simulink library "truetime"  (R2012a)
settings: Solver=ode45  SolverMode=SingleTasking  StartTime=0.0  StopTime=10.0  RelTol=1e-3
undefined symbols (not defined in the file or in its folder): sfunchk
settings Model: ExtModeAutoUpdateStatusClock=off  Creator=dan  LastModifiedBy=AC

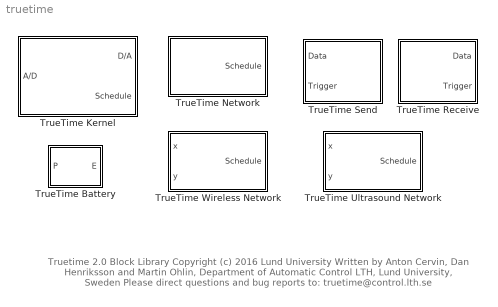
== system truetime ==
  note: Truetime 2.0  Block Library
      | Copyright (c) 2016 Lund University
      | Written by Anton Cervin, Dan Henriksson and Martin Ohlin,
      | Department of Automatic Control LTH, Lund University, Sweden
      | Please direct questions and bug reports to:  truetime@control.lth.se
  TrueTime Battery : Subsystem  mask{energy=1}
      mask prompts: energy "Initial energy:"
  TrueTime Kernel : Subsystem  InitFcn=sfunchk(get_param(gcb,'sfun'));  mask{sfun=node_init, args=[], ninputsoutputs=[1 1], ntriggers=0, trigtype=falling, nwnodenbr=[], clockoffsetdrift=[0 0], schedoutput=on, battery=off, poweroutput=off, label=}
      mask prompts: sfun "Name of init function (MEX or MATLAB):"; args "Init function argument (arbitrary struct):"; ninputsoutputs "Number of analog inputs and outputs:"; ntriggers "Number of external triggers:"; trigtype "Trigger type:"; nwnodenbr "(Network and) Node number(s):"; clockoffsetdrift "Local clock offset and drift:"; schedoutput "Show Schedule output port"; battery "Show Energy supply input port"; poweroutput "Show Power consumption output port"
      mask init:
      | ttkernel_callback(gcb,{sfun,args,ninputsoutputs,ntriggers,trigtype,nwnodenbr,clockoffsetdrift,schedoutput,battery,poweroutput})
      settings: ErrorFcn=ttkernel_error
      mask StyleString: edit,edit,edit,edit,popup(rising|falling|either),edit,edit,checkbox,checkbox,checkbox,edit
      mask Display: disp(get_param(gcb,'label'))
  TrueTime Network : Subsystem  mask(Real-Time Network){nwtype=CSMA/CD (Ethernet), nwnbr=1, nnodes=1, rate=10000000, minsize=512, lossprob=0, seed=0, bandwidths=[0.5 0.5], slotsize=512, schedule=[1 1 2], memsize=80000, buftype=Common buffer, overflow=Retransmit, dynSchedule=0, miniSlotSize=0, NIT=0, QSortMode=FIFO, sync=0, irtSchedule=0, nrtLength=0, nodeGraph=0, scheduleoutput=on}
      mask prompts: nwtype "Network type:"; nwnbr "Network number:"; nnodes "Number of nodes:"; rate "Data rate (bits/s):"; minsize "Minimum frame size (bits):"; lossprob "Loss probability (0-1):"; seed "Initial seed:"; bandwidths "Bandwidth allocations:"; slotsize "Slotsize (bits):"; schedule "Static schedule:"; memsize "Total switch memory (bits):"; buftype "Switch buffer type:"; overflow "Switch overflow behavior:"; dynSchedule "Dynamic Schedule:"; miniSlotSize "Mini slot size (bits):"; NIT "Network idle time (bits):"; QSortMode "Input Queue Sorted by:"; sync "Synchronization length (bits):"; irtSchedule "IRT Schedule [msgID from to start arrival]:"; nrtLength "RT Class 1/NRT length (bits):"; nodeGraph "Node connection graph (nbrOfnodes x nbrOfNodes):"; scheduleoutput "Show Schedule output port:"
      mask init:
      | ttnetwork_callback(gcb,nwnbr,nnodes,scheduleoutput)
      mask StyleString: popup(CSMA/CD (Ethernet)|CSMA/AMP (CAN)|Round Robin|FDMA|TDMA|Switched Ethernet|FlexRay|PROFINET|NCM),edit,edit,edit,edit,edit,edit,edit,edit,edit,edit,popup(Common buffer|Symmetric output buffers),popup(Retransmit|Drop),edit,edit,edit,popup(FIFO|Priority),edit,edit,edit,edit,checkbox
      mask CallbackString: ttnetwork_callback|||||||||||||||||||||
      mask Display: disp(nwnbr)
  TrueTime Receive : Subsystem  mask{nwnbr=1, receiver=1, outdim=1, triggeroutput=on, senderoutput=off, lengthoutput=off, priorityoutput=off, timestampoutput=off, signalpoweroutput=off, msgIDoutput=off}
      mask prompts: nwnbr "Network number:"; receiver "Receiver id:"; outdim "Data output port dimension:"; triggeroutput "Show trigger output port"; senderoutput "Show sender output port"; lengthoutput "Show length output port"; priorityoutput "Show priority output port"; timestampoutput "Show timestamp output port"; signalpoweroutput "Show signal power output port"; msgIDoutput "Show message id output port"
      mask init:
      | ttreceive_callback(gcb,nwnbr,receiver,triggeroutput,senderoutput,lengthoutput,priorityoutput,timestampoutput,signalpoweroutput,msgIDoutput)
      mask Display: disp([num2str(nwnbr) ': ' num2str(receiver)])
  TrueTime Send : Subsystem  mask{trigger=falling, nwnbr=1, sender=1, indim=1, recsource=internal, receiver=1, lengthsource=internal, length=1000, priosource=internal, prio=1, msgIDsource=internal, msgID=0, dynamicSegment=Dynamic}
      mask prompts: trigger "Trigger type:"; nwnbr "Network number:"; sender "Sender id:"; indim "Data input port dimension:"; recsource "Receiver source:"; receiver "Receiver id:"; lengthsource "Length source:"; length "Data length (bits):"; priosource "Priority source:"; prio "Priority (for CAN):"; msgIDsource "Message ID source:"; msgID "Message ID:"; dynamicSegment "Segment (for FlexRay):"
      mask init:
      | ttsend_callback(gcb,trigger,nwnbr,sender,recsource,lengthsource,priosource,msgIDsource)
      mask StyleString: popup(rising|falling|either),edit,edit,edit,popup(internal|external),edit,popup(internal|external),edit,popup(internal|external),edit,popup(internal|external),edit,popup(static|dynamic)
      mask CallbackString: ||||ttsend_callback||ttsend_callback||ttsend_callback||ttsend_callback||
      mask Display: disp([num2str(nwnbr) ': ' num2str(sender)])
  TrueTime Ultrasound Network : Subsystem  mask(Ultrasound Network){nwnbr=1, nnodes=1, reach=10.0, pinglength=0.001, speedofsound=344.0, scheduleoutput=on}
      mask prompts: nwnbr "Network Number:"; nnodes "Number of nodes:"; reach "Reach (m):"; pinglength "Ping length (s):"; speedofsound "Speed of sound (m/s):"; scheduleoutput "Show schedule output port"
      mask init:
      | ttusnetwork_callback(gcb,{nwnbr,nnodes,reach,pinglength,speedofsound,scheduleoutput})
      mask Display: disp(nwnbr)
  TrueTime Wireless Network : Subsystem  mask(Wireless Network){nwtype=802.11b (WLAN), nwnbr=1, nnodes=2, rate=800000, minsize=272, transpower=20, threshold=-48, use_pathloss_function=default, pathloss=3.5, pathloss_function=, acktimeout=0.00004, retrylimit=5, error_threshold=0.03, lossprob=0, seed=0, scheduleoutput=on, poweroutput=off}
      mask prompts: nwtype "Network type:"; nwnbr "Network Number:"; nnodes "Number of nodes:"; rate "Data rate (bits/s):"; minsize "Minimum frame size (bits):"; transpower "Transmit power (dbm):"; threshold "Receiver signal threshold (dbm):"; use_pathloss_function "Pathloss function:"; pathloss "Pathloss exponent (1/distance^x):"; pathloss_function "Matlab pathloss function:"; acktimeout "ACK timeout (s):"; retrylimit "Retry limit:"; error_threshold "Error coding threshold:"; lossprob "Loss probability (0-1):"; seed "Initial seed:"; scheduleoutput "Show Schedule output port"; poweroutput "Show Power consumption output port"
      mask init:
      | ttwnetwork_callback(gcb,{nwtype,nwnbr,nnodes,rate,minsize,transpower,threshold,use_pathloss_function,pathloss,pathloss_function,acktimeout,retrylimit,error_threshold,lossprob,seed,scheduleoutput,poweroutput})
      mask StyleString: popup(802.11b (WLAN)|802.15.4 (ZigBee)|NCM_WIRELESS),edit,edit,edit,edit,edit,edit,popup(default|custom),edit,edit,edit,edit,edit,edit,edit,checkbox,checkbox
      mask CallbackString: |||||||ttwnetwork_callback|||||||||
      mask Display: disp(nwnbr)

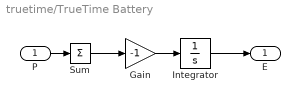
== system truetime/TrueTime Battery ==
  P : Inport
  Gain : Gain  Gain=-1  SaturateOnIntegerOverflow=on  OutDataTypeStr=Inherit: Same as input  ParamDataTypeStr=Inherit: Same as input
  Integrator : Integrator  InitialCondition=energy  LimitOutput=on  UpperSaturationLimit=energy  LowerSaturationLimit=0
  Sum : Sum  Inputs=1  SaturateOnIntegerOverflow=on  InputSameDT=on  OutDataTypeStr=Inherit: Same as first input
  E : Outport
  wires:
  Integrator/1 -> E/1
  Gain/1 -> Integrator/1
  P/1 -> Sum/1
  Sum/1 -> Gain/1

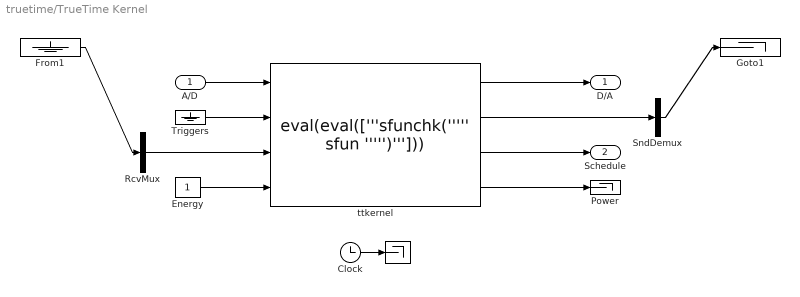
== system truetime/TrueTime Kernel ==
  A/D : Inport
  " " : Terminator
  Clock : Clock
  Energy : Constant
  From1 : Ground
  Goto1 : Terminator
  Power : Terminator
  RcvMux : Mux  Inputs=1
  SndDemux : Demux  Outputs=1
  Triggers : Ground
  ttkernel : S-Function  FunctionName=eval(eval(['''sfunchk(''''' sfun ''''')''']))  Parameters=sfun, args, ninputsoutputs, ntriggers, trigtype, nwnodenbr, clockoffsetdrift  EnableBusSupport=off
  D/A : Outport
  Schedule : Outport  Port=2
  wires:
  ttkernel/4 -> Power/1
  Energy/1 -> ttkernel/4
  A/D/1 -> ttkernel/1
  ttkernel/2 -> SndDemux/1
  ttkernel/1 -> D/A/1
  ttkernel/3 -> Schedule/1
  Triggers/1 -> ttkernel/2
  RcvMux/1 -> ttkernel/3
  Clock/1 -> " "/1
  From1/1 -> RcvMux/1
  SndDemux/1 -> Goto1/1

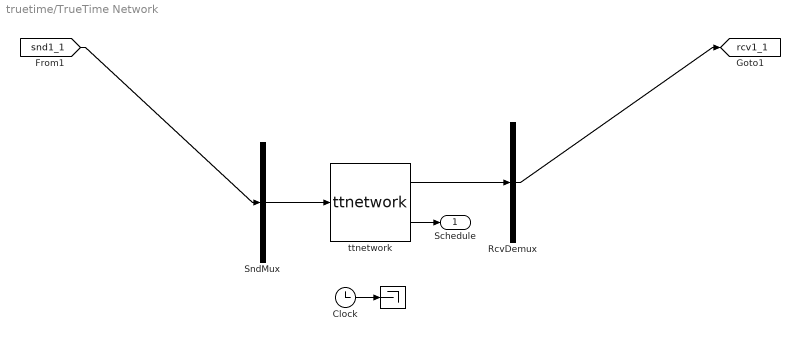
== system truetime/TrueTime Network ==
  " " : Terminator
  Clock : Clock
  RcvDemux : Demux  Outputs=1
  SndMux : Mux  Inputs=1
  ttnetwork : S-Function  FunctionName=ttnetwork  Parameters=nwtype,nwnbr,nnodes,rate,minsize,lossprob,bandwidths,slotsize,schedule,memsize,buftype,overflow,seed,dynSchedule,miniSlotSize,NIT,QSortMode,sync,irtSchedule,nrtLength,nodeGraph  EnableBusSupport=off
  Schedule : Outport
  tag scope: rcv1_1=global
  wires:
  ttnetwork/2 -> Schedule/1
  ttnetwork/1 -> RcvDemux/1
  SndMux/1 -> ttnetwork/1
  Clock/1 -> " "/1
  [snd1_1] -> SndMux/1
  RcvDemux/1 -> [rcv1_1]

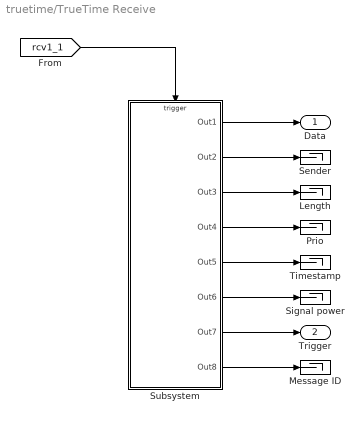
== system truetime/TrueTime Receive ==
  Length : Terminator
  Message ID : Terminator
  Prio : Terminator
  Sender : Terminator
  Signal power : Terminator
  Subsystem : Subsystem  TreatAsAtomicUnit=on
  Timestamp : Terminator
  Data : Outport
  Trigger : Outport  Port=2
  wires:
  Subsystem/8(Out8) -> Message ID/1
  Subsystem/1(Out1) -> Data/1
  Subsystem/3(Out3) -> Length/1
  Subsystem/2(Out2) -> Sender/1
  Subsystem/4(Out4) -> Prio/1
  [rcv1_1] -> Subsystem/Trigger
  Subsystem/5(Out5) -> Timestamp/1
  Subsystem/7(Out7) -> Trigger/1
  Subsystem/6(Out6) -> Signal power/1

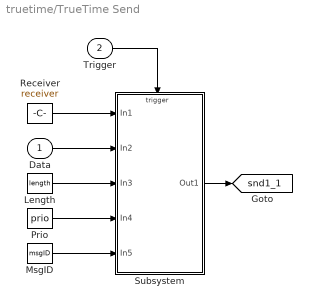
== system truetime/TrueTime Send ==
  Data : Inport
  Trigger : Inport  Port=2
  Length : Constant  Value=length
  MsgID : Constant  Value=msgID
  Prio : Constant  Value=prio
  Receiver : Constant  Value=receiver
  Subsystem : Subsystem  TreatAsAtomicUnit=on
  tag scope: snd1_1=global
  wires:
  MsgID/1 -> Subsystem/5(In5)
  Trigger/1 -> Subsystem/Trigger
  Subsystem/1(Out1) -> [snd1_1]
  Data/1 -> Subsystem/2(In2)
  Receiver/1 -> Subsystem/1(In1)
  Length/1 -> Subsystem/3(In3)
  Prio/1 -> Subsystem/4(In4)

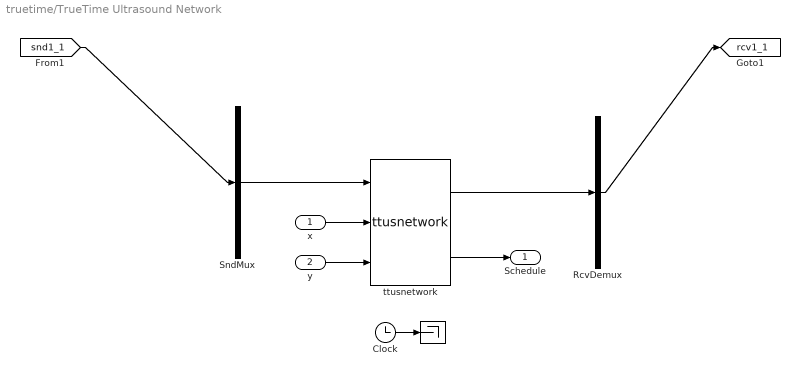
== system truetime/TrueTime Ultrasound Network ==
  x : Inport
  y : Inport  Port=2
  " " : Terminator
  Clock : Clock
  RcvDemux : Demux  Outputs=1
  SndMux : Mux  Inputs=1
  ttusnetwork : S-Function  FunctionName=ttusnetwork  Parameters=nwnbr,nnodes,reach,pinglength,speedofsound  EnableBusSupport=off
  Schedule : Outport
  tag scope: rcv1_1=global
  wires:
  SndMux/1 -> ttusnetwork/1
  ttusnetwork/1 -> RcvDemux/1
  ttusnetwork/2 -> Schedule/1
  x/1 -> ttusnetwork/2
  y/1 -> ttusnetwork/3
  Clock/1 -> " "/1
  [snd1_1] -> SndMux/1
  RcvDemux/1 -> [rcv1_1]

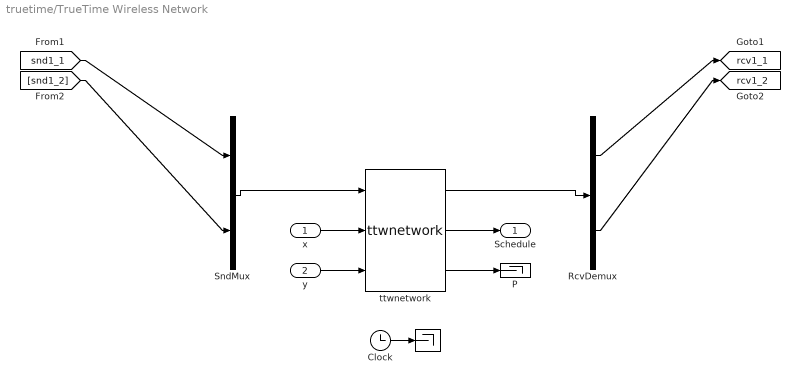
== system truetime/TrueTime Wireless Network ==
  x : Inport
  y : Inport  Port=2
  " " : Terminator
  Clock : Clock
  P : Terminator
  RcvDemux : Demux  Outputs=2
  SndMux : Mux  Inputs=2
  ttwnetwork : S-Function  FunctionName=ttwnetwork  Parameters=nwtype,nwnbr,nnodes,rate,minsize,transpower,threshold,pathloss,use_pathloss_function,pathloss_function,acktimeout,retrylimit,error_threshold,lossprob,seed  EnableBusSupport=off
  Schedule : Outport
  tag scope: rcv1_1=global, rcv1_2=global
  wires:
  ttwnetwork/3 -> P/1
  SndMux/1 -> ttwnetwork/1
  ttwnetwork/1 -> RcvDemux/1
  ttwnetwork/2 -> Schedule/1
  x/1 -> ttwnetwork/2
  y/1 -> ttwnetwork/3
  Clock/1 -> " "/1
  [snd1_1] -> SndMux/1
  [snd1_2] -> SndMux/2
  RcvDemux/1 -> [rcv1_1]
  RcvDemux/2 -> [rcv1_2]

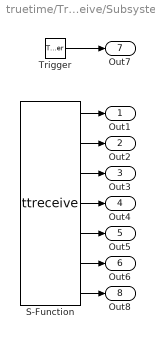
== system truetime/TrueTime Receive/Subsystem ==
  Trigger : TriggerPort  TriggerType=either  ShowOutputPort=on
  S-Function : S-Function  FunctionName=ttreceive  Parameters=nwnbr,receiver,outdim  EnableBusSupport=off
  Out1 : Outport
  Out2 : Outport  Port=2
  Out3 : Outport  Port=3
  Out4 : Outport  Port=4
  Out5 : Outport  Port=5
  Out6 : Outport  Port=6
  Out7 : Outport  Port=7
  Out8 : Outport  Port=8
  wires:
  S-Function/7 -> Out8/1
  S-Function/1 -> Out1/1
  S-Function/2 -> Out2/1
  S-Function/3 -> Out3/1
  S-Function/4 -> Out4/1
  S-Function/5 -> Out5/1
  S-Function/6 -> Out6/1
  Trigger/1 -> Out7/1

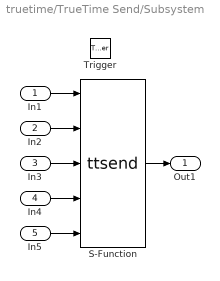
== system truetime/TrueTime Send/Subsystem ==
  In1 : Inport
  In2 : Inport  Port=2
  In3 : Inport  Port=3
  In4 : Inport  Port=4
  In5 : Inport  Port=5
  Trigger : TriggerPort  TriggerType=falling
  S-Function : S-Function  FunctionName=ttsend  Parameters=nwnbr,sender,indim,dynamicSegment  EnableBusSupport=off
  Out1 : Outport
  wires:
  In5/1 -> S-Function/5
  In4/1 -> S-Function/4
  In3/1 -> S-Function/3
  S-Function/1 -> Out1/1
  In2/1 -> S-Function/2
  In1/1 -> S-Function/1
